simulink model "frft_design"  (R2025a)
settings: Solver=VariableStepAuto  StartTime=0.0  StopTime=10.0  RelTol=1e-3
libraries: hdlBasic x20
settings Model: Creator=daniel  LastModifiedBy=daniel

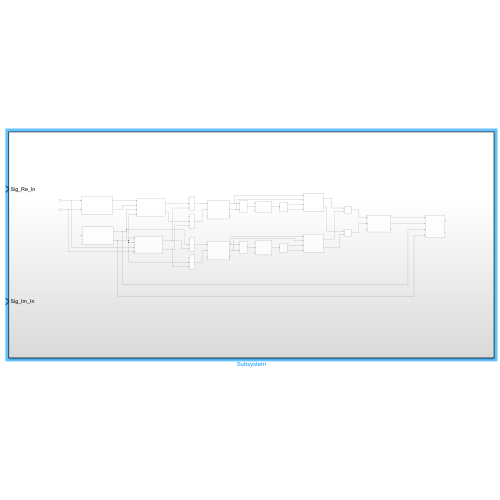
[thumbnail: Simulink's stored preview of the top-level diagram]
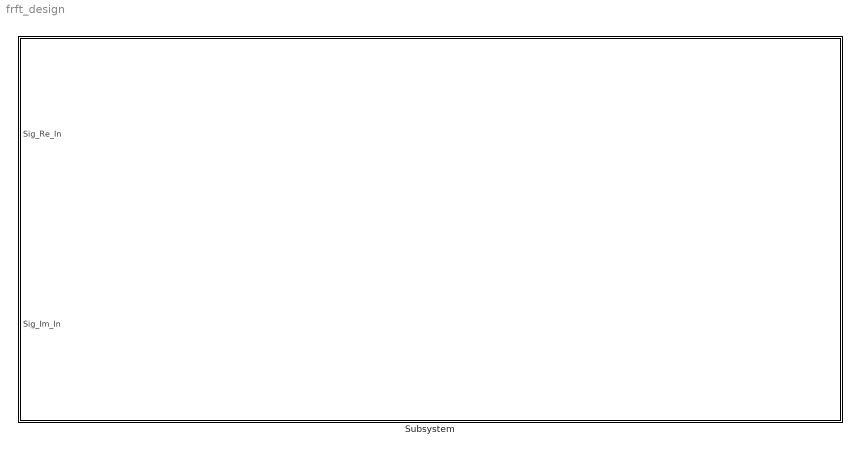
== system frft_design ==
  Subsystem : Subsystem

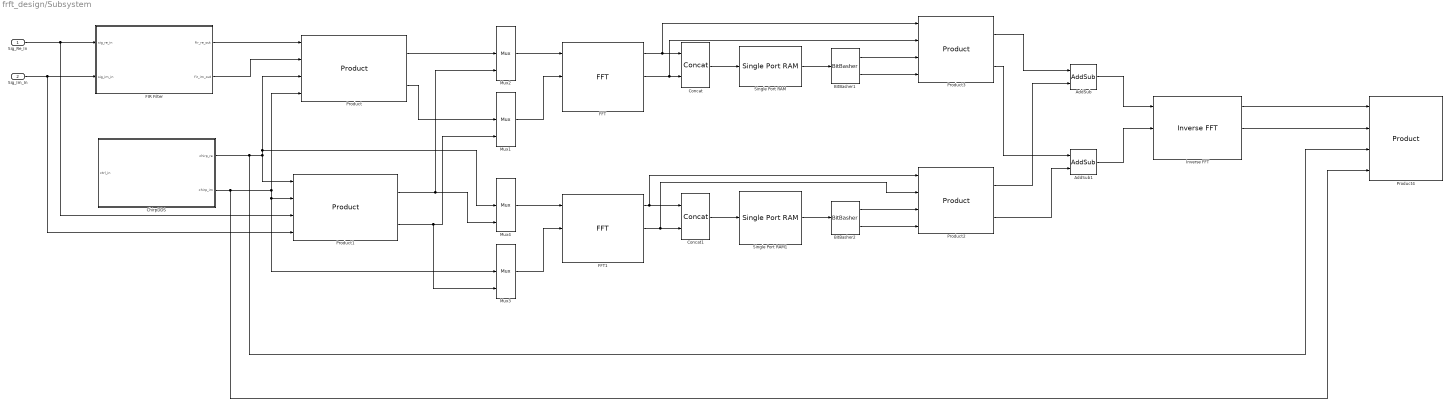
== system frft_design/Subsystem ==
  Sig_Re_In : Inport
  Sig_Im_In : Inport  Port=2
  AddSub : hdlBasic/AddSub  mode=Addition  use_carryin=off  use_carryout=off  en=off  latency=1  precision=Full  arith_type=Unsigned  n_bits=16  bin_pt=14  quantization=Truncate  overflow=Wrap  use_behavioral_HDL=off  hw_selection=Fabric  pipelined=off  XmcBlockStatus=1  maskContainerNames=tabcontainer1  block_type=addsub  block_config=sysgen:Addsub_config
  AddSub1 : hdlBasic/AddSub  mode=Addition  use_carryin=off  use_carryout=off  en=off  latency=1  precision=Full  arith_type=Unsigned  n_bits=16  bin_pt=14  quantization=Truncate  overflow=Wrap  use_behavioral_HDL=off  hw_selection=Fabric  pipelined=off  XmcBlockStatus=1  maskContainerNames=tabcontainer1  block_type=addsub  block_config=sysgen:Addsub_config
  BitBasher1 : hdlBasic/BitBasher  bitexpr=|  display_expr=off  sr_1=d_re  arith_type1=Unsigned  bin_pt1=0  sr_2=d_im  arith_type2=Unsigned  bin_pt2=0  sr_3=3  arith_type3=Unsigned  bin_pt3=0  sr_4=4  arith_type4=Unsigned  bin_pt4=0  XmcBlockStatus=1  maskContainerNames=group1  block_type=bitbasher  block_config=sysgen:BitBasher_config
      | d_re={d}
      | d_im={d}
  BitBasher2 : hdlBasic/BitBasher  bitexpr=|  display_expr=off  sr_1=d_re  arith_type1=Unsigned  bin_pt1=0  sr_2=d_im  arith_type2=Unsigned  bin_pt2=0  sr_3=3  arith_type3=Unsigned  bin_pt3=0  sr_4=4  arith_type4=Unsigned  bin_pt4=0  XmcBlockStatus=1  maskContainerNames=group1  block_type=bitbasher  block_config=sysgen:BitBasher_config
      | d_re={d}
      | d_im={d}
  ChirpDDS : Subsystem
  Concat : hdlBasic/Concat  num_inputs=2  XmcBlockStatus=1  maskContainerNames=group1  block_type=concat  block_config=sysgen:Concat_config
  Concat1 : hdlBasic/Concat  num_inputs=2  XmcBlockStatus=1  maskContainerNames=group1  block_type=concat  block_config=sysgen:Concat_config
  FFT : hdlBasic/FFT  transform_length=1024  scale_result_by_fft_length=off  bit_reversed_order=off  optimizegoal=Performance  start_frame=on  simulation_type=fast_sim  simulation_model=sysgen:ForwardFFT_Macro  latency=1  XmcBlockStatus=1  maskContainerNames=group1  block_type=xfft_forward  block_config=sysgen:FFTMacro_config
  FFT1 : hdlBasic/FFT  transform_length=1024  scale_result_by_fft_length=off  bit_reversed_order=off  optimizegoal=Performance  start_frame=on  simulation_type=fast_sim  simulation_model=sysgen:ForwardFFT_Macro  latency=1  XmcBlockStatus=1  maskContainerNames=group1  block_type=xfft_forward  block_config=sysgen:FFTMacro_config
  FIR Filter : Subsystem
  Inverse FFT : hdlBasic/Inverse FFT  transform_length=1024  scale_result_by_fft_length=off  bit_reversed_order=off  optimizegoal=Performance  start_frame=on  simulation_type=fast_sim  simulation_model=sysgen:InverseFFT_Macro  latency=1  XmcBlockStatus=1  maskContainerNames=group1  block_type=xfft_inverse  block_config=sysgen:Inverse_FFTMacro_config
  Mux{1..4} (4 alike) : hdlBasic/Mux  inputs=2  en=off  latency=1  precision=Full  arith_type=Unsigned  n_bits=16  bin_pt=14  quantization=Truncate  overflow=Wrap  XmcBlockStatus=1  maskContainerNames=tabcontainer1  block_type=mux  block_config=sysgen:Mux_config
  Product{,1..4} (5 alike) : hdlBasic/Product  complex_multiplier=on  optimizegoal=Performance  simulation_type=fast_sim  simulation_model=sysgen:product_macro  XmcBlockStatus=1  maskContainerNames=<empty>  block_type=product_macro  block_config=sysgen:ProductMacro_config
  Single Port RAM : hdlBasic/Single Port RAM  depth=16  initVector=sin(pi*(0:15)/16)  distributed_mem=Block RAM  write_mode=Read After Write  rst=off  init_reg=0  en=off  optimize_latency=off  latency=1  optimize=Area  dbl_ovrd=off  simulation_type=fast_sim  XmcBlockStatus=1  maskContainerNames=tabcontainer1  block_type=spram  block_config=sysgen:SPRAM_config
  Single Port RAM1 : hdlBasic/Single Port RAM  depth=16  initVector=sin(pi*(0:15)/16)  distributed_mem=Block RAM  write_mode=Read After Write  rst=off  init_reg=0  en=off  optimize_latency=off  latency=1  optimize=Area  dbl_ovrd=off  simulation_type=fast_sim  XmcBlockStatus=1  maskContainerNames=tabcontainer1  block_type=spram  block_config=sysgen:SPRAM_config
  wires:
  ? -> ChirpDDS/1(ctrl_in)
  FFT/1 -> Concat/1, Product3/1
  FFT/2 -> Concat/2, Product3/2
  Concat/1 -> Single Port RAM/2
  FFT1/1 -> Product2/1, Concat1/1
  FFT1/2 -> Product2/2, Concat1/2
  Single Port RAM/1 -> BitBasher1/1
  ChirpDDS/2(chirp_im) -> Product4/4, Mux3/2, Product1/2, Product/4
  FIR Filter/1(fir_re_out) -> Product/1
  FIR Filter/2(fir_im_out) -> Product/2
  Mux2/1 -> FFT/1
  Mux1/1 -> FFT/2
  Product/1 -> Mux2/2
  Product1/1 -> Mux4/3, Mux2/3
  Product/2 -> Mux1/2
  Product1/2 -> Mux1/3, Mux3/3
  Mux4/1 -> FFT1/1
  Mux3/1 -> FFT1/2
  Sig_Re_In/1 -> Product1/3, FIR Filter/1(sig_re_in)
  Sig_Im_In/1 -> Product1/4, FIR Filter/2(sig_im_in)
  Concat1/1 -> Single Port RAM1/2
  Single Port RAM1/1 -> BitBasher2/1
  Product3/1 -> AddSub/1
  Product2/1 -> AddSub/2
  Product3/2 -> AddSub1/1
  Product2/2 -> AddSub1/2
  AddSub1/1 -> Inverse FFT/2
  AddSub/1 -> Inverse FFT/1
  BitBasher1/1 -> Product3/3
  BitBasher1/2 -> Product3/4
  BitBasher2/1 -> Product2/3
  BitBasher2/2 -> Product2/4
  Inverse FFT/1 -> Product4/1
  Inverse FFT/2 -> Product4/2
  ChirpDDS/1(chirp_re) -> Product1/1, Product/3, Mux4/2, Product4/3

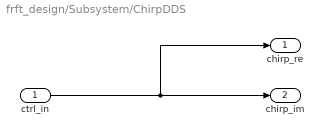
== system frft_design/Subsystem/ChirpDDS ==
  ctrl_in : Inport
  chirp_re : Outport
  chirp_im : Outport  Port=2
  wires:
  ctrl_in/1 -> chirp_im/1, chirp_re/1

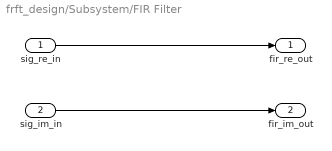
== system frft_design/Subsystem/FIR Filter ==
  sig_re_in : Inport
  sig_im_in : Inport  Port=2
  fir_re_out : Outport
  fir_im_out : Outport  Port=2
  wires:
  sig_re_in/1 -> fir_re_out/1
  sig_im_in/1 -> fir_im_out/1
